simulink model "Cntrl200plant"  (R2017a)
settings: Solver=VariableStepAuto  StartTime=0.0  StopTime=10.0  RelTol=1e-3
settings Model: Creator=Dell  LastModifiedBy=Dell

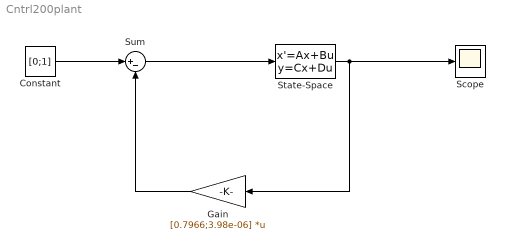
== system Cntrl200plant ==
  Constant : Constant  Value=[0;1]  VectorParams1D=off
  Gain : Gain  Gain=[0.7966;3.98e-06]  Multiplication=Matrix(K*u)
  Scope : Scope
  State-Space : StateSpace  A="[-0.003401570000000  -0.000000016230000; 1 0]"  B=[1;0]  C=[1 0]  D=[0]  X0="[0  0]"
  Sum : Sum  Inputs=|+-
  wires:
  Sum/1 -> State-Space/1
  State-Space/1 -> Scope/1, Gain/1
  Gain/1 -> Sum/2
  Constant/1 -> Sum/1
